simulink model "KeplerianPropagator_Basic2"  (R2017b)
settings: Solver=FixedStepAuto  StartTime=0.0  StopTime=stopTime  FixedStep=stepSize  RelTol=1e-3
values from neighbouring files (symbols this model uses):
  a = (mu/n^2)^(1/3)    [TLE_Reader.m]
  e = L3(1,5)/1e7    [TLE_Reader.m]
  inc = L3(1,3)    [TLE_Reader.m]
  M0 = M    [AA279D_PSET1.m]    (also in AA279D_PSET2.m; AA279D_PSET2_a_change.m)
  n = revs_per_day*2*pi/(24*3600)    [TLE_Reader.m]
  RAAN = L3(1,4)    [TLE_Reader.m]
  tol = 10^-5    (= 1e-05)    [AA279D_PSET1.m]    (also in AA279D_PSET2.m; AA279D_PSET2_a_change.m)
  w = L3(1,6)    [TLE_Reader.m]
libraries: simulink_extras x4
settings Model: Creator=cwcovert  LastModifiedBy=cwcovert

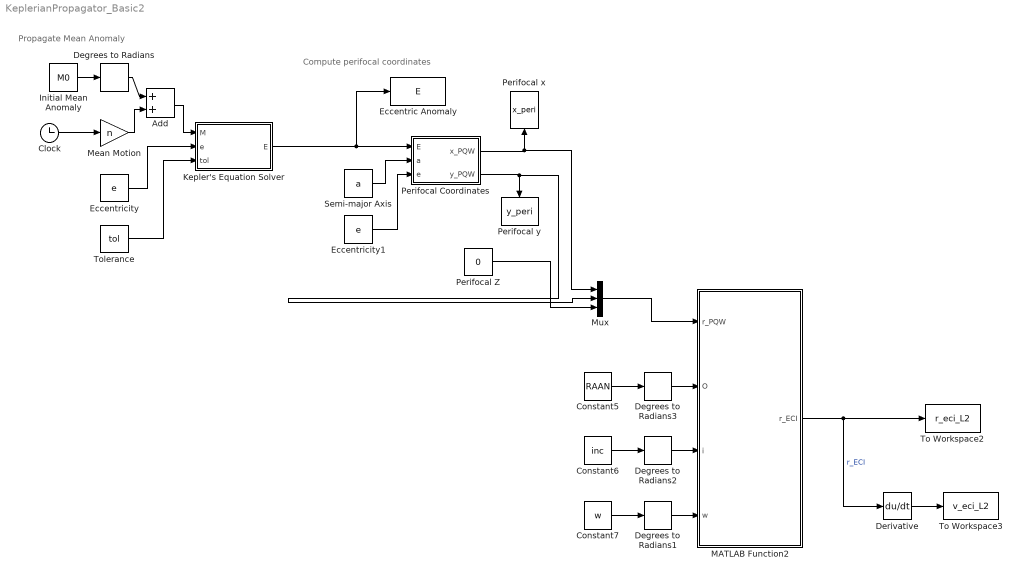
== system KeplerianPropagator_Basic2 ==
  note: Propagate Mean Anomaly
  note: Compute perifocal coordinates
  Add : Sum
  Clock : Clock
  Constant5 : Constant  Value=RAAN
  Constant6 : Constant  Value=inc
  Constant7 : Constant  Value=w
  Degrees to Radians{,1..3} (4 alike) : simulink_extras/Transformations/Degrees to Radians
  Derivative : Derivative
  Eccentric Anomaly : ToWorkspace  VariableName=E  SampleTime=-1
  Eccentricity : Constant  Value=e
  Eccentricity1 : Constant  Value=e
  Initial Mean Anomaly : Constant  Value=M0
  Kepler's Equation Solver : MATLAB Function  TreatAsAtomicUnit=on
  MATLAB Function2 : MATLAB Function  TreatAsAtomicUnit=on
  Mean Motion : Gain  Gain=n
  Mux : Mux  Inputs=3
  Perifocal Coordinates : MATLAB Function  TreatAsAtomicUnit=on
  Perifocal Z : Constant  Value=0
  Perifocal x : ToWorkspace  VariableName=x_peri  SampleTime=-1
  Perifocal y : ToWorkspace  VariableName=y_peri  SampleTime=-1
  Semi-major Axis : Constant  Value=a
  To Workspace2 : ToWorkspace  VariableName=r_eci_L2  SampleTime=-1
  To Workspace3 : ToWorkspace  VariableName=v_eci_L2  SampleTime=-1
  Tolerance : Constant  Value=tol
  wires:
  Perifocal Z/1 -> Mux/3
  Mean Motion/1 -> Add/2
  Tolerance/1 -> Kepler's Equation Solver/3(tol)
  Kepler's Equation Solver/1(E) -> Perifocal Coordinates/1(E), Eccentric Anomaly/1
  Semi-major Axis/1 -> Perifocal Coordinates/2(a)
  Add/1 -> Kepler's Equation Solver/1(M)
  Clock/1 -> Mean Motion/1
  Perifocal Coordinates/1(x_PQW) -> Mux/1, Perifocal x/1
  Initial Mean Anomaly/1 -> Degrees to Radians/1
  Perifocal Coordinates/2(y_PQW) -> Mux/2, Perifocal y/1
  Degrees to Radians/1 -> Add/1
  Eccentricity1/1 -> Perifocal Coordinates/3(e)
  Eccentricity/1 -> Kepler's Equation Solver/2(e)
  MATLAB Function2/1(r_ECI) -> Derivative/1, To Workspace2/1  "r_ECI"
  Degrees to Radians1/1 -> MATLAB Function2/4(w)
  Degrees to Radians3/1 -> MATLAB Function2/2(O)
  Constant5/1 -> Degrees to Radians3/1
  Constant7/1 -> Degrees to Radians1/1
  Derivative/1 -> To Workspace3/1
  Degrees to Radians2/1 -> MATLAB Function2/3(i)
  Constant6/1 -> Degrees to Radians2/1
  Mux/1 -> MATLAB Function2/1(r_PQW)

== matlab function KeplerianPropagator_Basic2/Kepler's Equation Solver ==
  data: M input; E output; e input; tol input
function E = MeanAnom2EccAnom(M, e, tol) 

% Compute eccentric anomaly from mean anomaly
%
% Inputs
% ------
% M         mean anomaly [rad]
% e         eccentricity
% tol       tolerance
%
% Outputs
% -------
% E         Eccentric anomaly [rad]
% v         velocity vector

% Check edge cases
if( M == pi || M == 0)
    E = M;
    return
end

% initial guess
if( M > pi )
    E = M - e/2;
else
    E = M + e/2;
end

err = 1;
count = 0;
while err > tol
    % Compute correction value
    delta = -(E - e*sin(E) - M)/(1 - e*cos(E));

    % Error
    err = abs(delta);
  
    E = E + delta;
    
    % Limit # of iterations
    count = count + 1;
    if count > 1e6
        return
    end
end

== matlab function KeplerianPropagator_Basic2/MATLAB Function2 ==
  data: r_PQW input; r_ECI output; O input; i input; w input
function r_ECI = PQW2ECI(r_PQW, O, i, w)

% Transform vector in perifocal to ECI
%
% Inputs
% ------
% r_PQW     position in perifocal coordinates
% i         inclination [rad]
% O       	right ascension of ascending node [rad]
% w         argument of pariapsis [rad]
%
% Outputs
% -------
% r_ECI     position in ECI coordinates

% Compute rotation matrix from PQW to ECI (3-1-3 Euler rots)
Rz_O = [cos(-O)     sin(-O)     0;
        -sin(-O)    cos(-O)     0;
        0           0           1;];
Rx_i = [1   0           0;
        0   cos(-i)     sin(-i);
        0   -sin(-i)    cos(-i);];
Rz_w = [cos(-w)     sin(-w)     0;
        -sin(-w)    cos(-w)     0;
        0           0           1;];
R_PWQ2ECI = Rz_O * Rx_i * Rz_w;

r_ECI = R_PWQ2ECI * r_PQW;

== matlab function KeplerianPropagator_Basic2/Perifocal Coordinates ==
  data: E input; a input; x_PQW output; e input; y_PQW output
function [x_PQW, y_PQW] = E2Pos(E, a, e)

% Compute position in perifocal coordinates
%
% Inputs
% ------
% E         Eccentric anomaly
% a         semi-major axis
%
% Outputs
% -------
% x         x position on orbital plane
% y         y position on orbital plane

% semi-latus rectum
p = a*(1 - e^2);

% Compute true anomaly from eccentric anomaly
cos_nu = (cos(E) - e) / (1 - e*cos(E));
sin_nu = (sin(E)*sqrt(1 - e^2)) / (1 - e*cos(E));
nu = atan2(sin_nu, cos_nu);

% Compute radial position
r = p / (1 + e*cos(nu));

% convert to cartesian
x_PQW = r*cos(nu);
y_PQW = r*sin(nu);
